simulink model "long"  (R2020a)
settings: Solver=VariableStepAuto  StartTime=0.0  StopTime=t_sim  MaxStep=0.01  RelTol=1e-3
values from neighbouring files (symbols this model uses):
  Cd0 = p_Cd(1)    [main.m]
  Cl0 = p_Cl(2)    [main.m]
  Cla = p_Cl(1)    [main.m]
  Cladot = pi + 2*pi*Gk/k    [main.m]
  Clde = Clde(1)    [main.m]
  Clq = -2*Cla*(h-3/4)    [main.m]
  Cm0 = p_Cm(2)    [main.m]
  Cma = p_Cm(1)    [main.m]
  Cmadot = pi*(h-1/2) + 2*pi*Gk/k*(h-1/4)    [main.m]
  Cmde = Clde(1)    [main.m]
  Cmq = -2*Cla*(h-1/2)^2    [main.m]
  delta_e = interp1(trim_polar(:,1),trim_polar(:,2),alpha)    [main.m]
  k = secante(func,0,1,1e-6,100)    [main.m]
  theta0 = 0    [main.m]
  u0 = tailsit.general.speed    [main.m]
  w0 = 0    [main.m]
undefined symbols (not defined in the file or in its folder): tailsit
libraries: simulink_extras x2
settings Model: Creator=willi  LastModifiedBy=willi
settings DataIOCC: ReturnWorkspaceOutputs=off
settings DebuggingCC: ArithmeticOperatorsInVariantConditions=warning
settings SFSimCC: SimUseLocalCustomCode=off  CustomCodeUndefinedFunction=UseInterfaceOnly
settings RTWCC: RTWUseLocalCustomCode=off

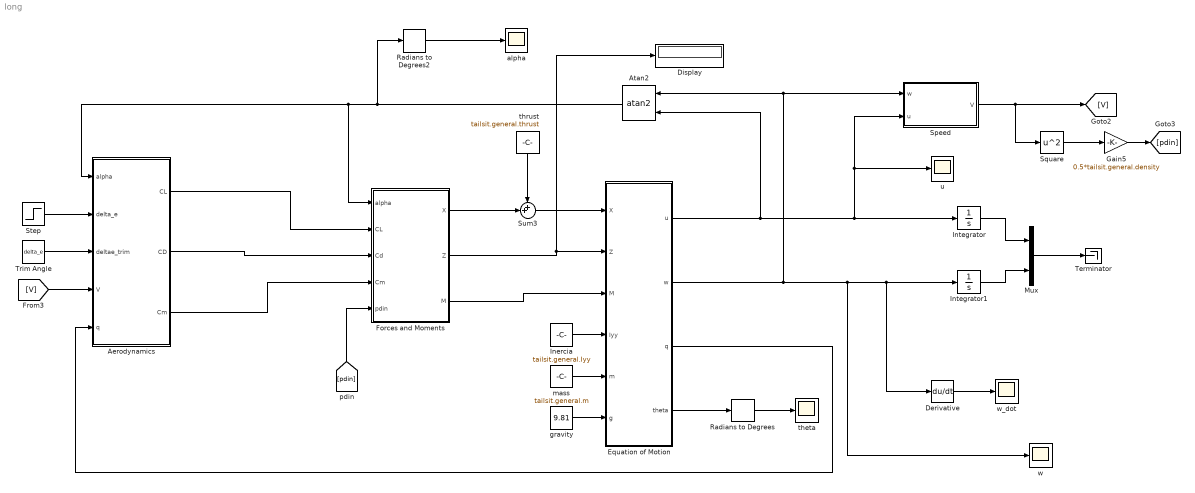
== system long ==
  Aerodynamics : Subsystem
  Atan2 : Trigonometry  Operator=atan2
  Derivative : Derivative
  Display : Display
  Equation of Motion : Subsystem  mask{initial_u=u0, initial_w=w0, initial_q=0.0, initial_theta=theta0}
      mask prompts: initial_u "Initial Speed (u, m/s)"; initial_w "Initial Speed (w, m/s)"; initial_q "Initial Angular Speed (q, rad/s)"; initial_theta "Euler Angle (theta, rad/s)"
  Forces and Moments : Subsystem  mask{area=tailsit.general.Sref, cref=tailsit.general.cbar}
      mask prompts: cref "Chord"
  Gain5 : Gain  Gain=0.5*tailsit.general.density
  Inercia : Constant  Value=tailsit.general.Iyy
  Integrator : Integrator
  Integrator1 : Integrator
  Mux : Mux  Inputs=2
  Radians to Degrees : simulink_extras/Transformations/Radians to Degrees
  Radians to Degrees2 : simulink_extras/Transformations/Radians to Degrees
  Speed : Subsystem
  Square : Math  Operator=square  SignedPower=on  SaturateOnIntegerOverflow=on
  Step : Step  Time=10  SampleTime=0
  Sum3 : Sum  Inputs=++|
  Terminator : Terminator
  Trim Angle : Constant  Value=delta_e
  alpha : Scope
  gravity : Constant  Value=9.81
  mass : Constant  Value=tailsit.general.m
  theta : Scope
  thrust : Constant  Value=tailsit.general.thrust
  u : Scope
  w : Scope
  w_dot : Scope
  wires:
  Forces and Moments/3(M) -> Equation of Motion/3(M)
  Forces and Moments/2(Z) -> Display/1, Equation of Motion/2(Z)
  Aerodynamics/1(CL) -> Forces and Moments/2(CL)
  thrust/1 -> Sum3/1
  Sum3/1 -> Equation of Motion/1(X)
  Forces and Moments/1(X) -> Sum3/2
  Equation of Motion/1(u) -> Integrator/1, Speed/2(u), u/1, Atan2/2
  Equation of Motion/2(w) -> Derivative/1, Integrator1/1, w/1, Speed/1("w "), Atan2/1
  Gain5/1 -> [pdin]
  [pdin] -> Forces and Moments/5(pdin)
  mass/1 -> Equation of Motion/5(m)
  gravity/1 -> Equation of Motion/6(g)
  Inercia/1 -> Equation of Motion/4(Iyy)
  Atan2/1 -> Radians to Degrees2/1, Aerodynamics/1(alpha), Forces and Moments/1(alpha)
  Radians to Degrees2/1 -> alpha/1
  Speed/1(V) -> [V], Square/1
  Square/1 -> Gain5/1
  Aerodynamics/2(CD) -> Forces and Moments/3(Cd)
  Aerodynamics/3(Cm) -> Forces and Moments/4(Cm)
  Trim Angle/1 -> Aerodynamics/3(deltae_trim)
  Equation of Motion/3(q) -> Aerodynamics/5(q)
  [V] -> Aerodynamics/4(V)
  Step/1 -> Aerodynamics/2(delta_e)
  Integrator/1 -> Mux/1
  Integrator1/1 -> Mux/2
  Mux/1 -> Terminator/1
  Derivative/1 -> w_dot/1
  Radians to Degrees/1 -> theta/1
  Equation of Motion/4(theta) -> Radians to Degrees/1

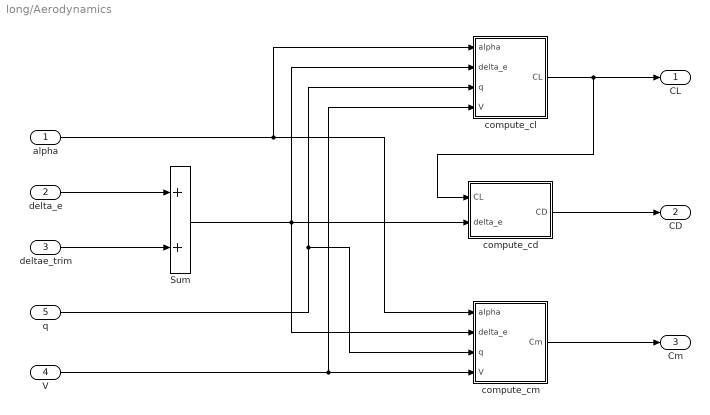
== system long/Aerodynamics ==
  alpha : Inport
  delta_e : Inport  Port=2
  deltae_trim : Inport  Port=3
  V : Inport  Port=4
  q : Inport  Port=5
  Sum : Sum
  compute_cd : Subsystem
  compute_cl : Subsystem
  compute_cm : Subsystem
  CL : Outport  VectorParamsAs1DForOutWhenUnconnected=off
  CD : Outport  Port=2  VectorParamsAs1DForOutWhenUnconnected=off
  Cm : Outport  Port=3  VectorParamsAs1DForOutWhenUnconnected=off
  wires:
  compute_cl/1(CL) -> compute_cd/1(CL), CL/1
  alpha/1 -> compute_cl/1(alpha), compute_cm/1(alpha)
  delta_e/1 -> Sum/1
  q/1 -> compute_cm/3(q), compute_cl/3(q)
  V/1 -> compute_cl/4(V), compute_cm/4(V)
  compute_cm/1(Cm) -> Cm/1
  compute_cd/1(CD) -> CD/1
  deltae_trim/1 -> Sum/2
  Sum/1 -> compute_cm/2(delta_e), compute_cl/2(delta_e), compute_cd/2(delta_e)

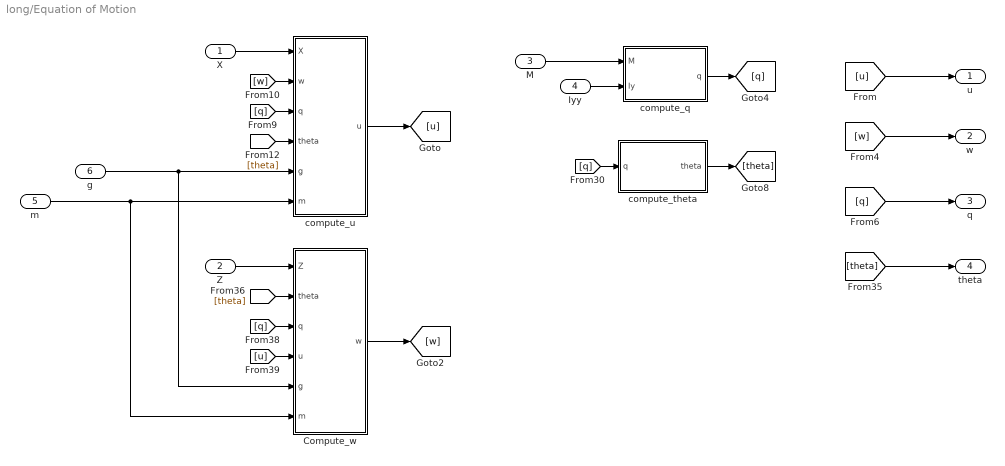
== system long/Equation of Motion ==
  X : Inport
  Z : Inport  Port=2
  M : Inport  Port=3
  Iyy : Inport  Port=4
  m : Inport  Port=5
  g : Inport  Port=6
  Compute_w : Subsystem
  compute_q : Subsystem
  compute_theta : Subsystem
  compute_u : Subsystem
  u : Outport  VectorParamsAs1DForOutWhenUnconnected=off
  w : Outport  Port=2  VectorParamsAs1DForOutWhenUnconnected=off
  q : Outport  Port=3  VectorParamsAs1DForOutWhenUnconnected=off
  theta : Outport  Port=4  VectorParamsAs1DForOutWhenUnconnected=off
  wires:
  X/1 -> compute_u/1(X)
  compute_u/1(u) -> [u]
  [u] -> u/1
  [w] -> w/1
  Z/1 -> Compute_w/1(Z)
  Compute_w/1(w) -> [w]
  M/1 -> compute_q/1(M)
  [q] -> q/1
  compute_q/1(q) -> [q]
  [w] -> compute_u/2(w)
  [q] -> compute_u/3(q)
  [theta] -> compute_u/4(theta)
  compute_theta/1("theta ") -> [theta]
  [q] -> compute_theta/1(q)
  [theta] -> theta/1
  [theta] -> Compute_w/2(theta)
  [q] -> Compute_w/3(q)
  [u] -> Compute_w/4(u)
  Iyy/1 -> compute_q/2(Iy)
  m/1 -> Compute_w/6(m), compute_u/6(m)
  g/1 -> Compute_w/5(g), compute_u/5(g)

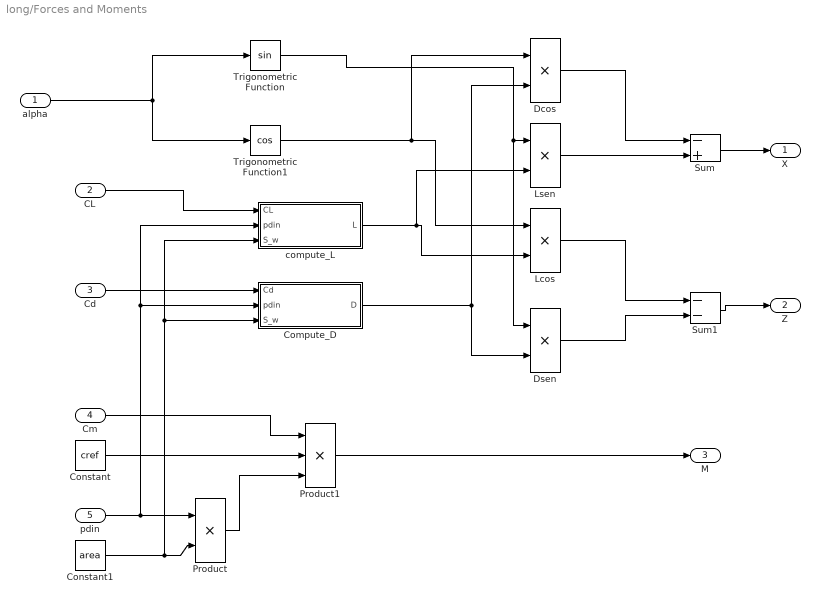
== system long/Forces and Moments ==
  alpha : Inport
  CL : Inport  Port=2
  Cd : Inport  Port=3
  Cm : Inport  Port=4
  pdin : Inport  Port=5
  Compute_D : Subsystem
  Constant : Constant  Value=cref
  Constant1 : Constant  Value=area
  Dcos : Product
  Dsen : Product
  Lcos : Product
  Lsen : Product
  Product : Product
  Product1 : Product  Inputs=3
  Sum : Sum  Inputs=-+
  Sum1 : Sum  Inputs=--
  Trigonometric Function : Trigonometry
  Trigonometric Function1 : Trigonometry  Operator=cos
  compute_L : Subsystem
  X : Outport  VectorParamsAs1DForOutWhenUnconnected=off
  Z : Outport  Port=2  VectorParamsAs1DForOutWhenUnconnected=off
  M : Outport  Port=3  VectorParamsAs1DForOutWhenUnconnected=off
  wires:
  Constant1/1 -> Compute_D/3(S_w), compute_L/3(S_w), Product/2
  Cm/1 -> Product1/1
  Constant/1 -> Product1/2
  Product/1 -> Product1/3
  Product1/1 -> M/1
  CL/1 -> compute_L/1(CL)
  Cd/1 -> Compute_D/1(Cd)
  pdin/1 -> Compute_D/2(pdin), compute_L/2(pdin), Product/1
  alpha/1 -> Trigonometric Function/1, Trigonometric Function1/1
  Sum/1 -> X/1
  Trigonometric Function1/1 -> Lcos/1, Dcos/1
  Compute_D/1(D) -> Dsen/2, Dcos/2
  compute_L/1(L) -> Lcos/2, Lsen/2
  Trigonometric Function/1 -> Dsen/1, Lsen/1
  Dcos/1 -> Sum/1
  Lsen/1 -> Sum/2
  Lcos/1 -> Sum1/1
  Dsen/1 -> Sum1/2
  Sum1/1 -> Z/1

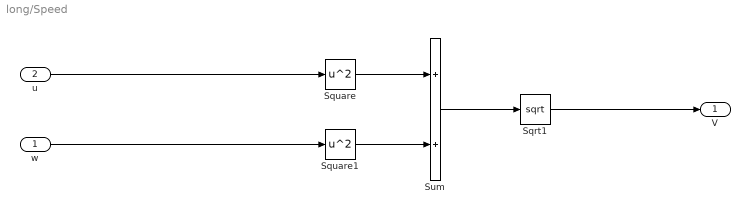
== system long/Speed ==
  "w " : Inport
  u : Inport  Port=2
  Sqrt1 : Sqrt  SaturateOnIntegerOverflow=on
  Square : Math  Operator=square  SignedPower=on  SaturateOnIntegerOverflow=on
  Square1 : Math  Operator=square  SignedPower=on  SaturateOnIntegerOverflow=on
  Sum : Sum
  V : Outport  VectorParamsAs1DForOutWhenUnconnected=off
  wires:
  Sum/1 -> Sqrt1/1
  Square1/1 -> Sum/2
  "w "/1 -> Square1/1
  Square/1 -> Sum/1
  u/1 -> Square/1
  Sqrt1/1 -> V/1

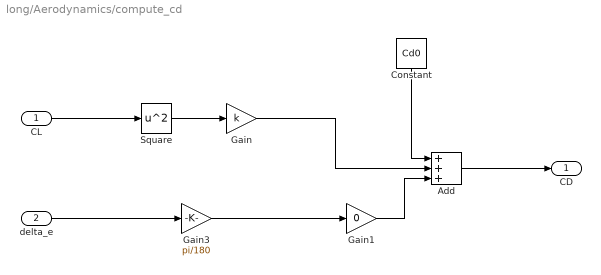
== system long/Aerodynamics/compute_cd ==
  CL : Inport
  delta_e : Inport  Port=2
  Add : Sum  Inputs=+++
  Constant : Constant  Value=Cd0
  Gain : Gain  Gain=k
  Gain1 : Gain  Gain=0
  Gain3 : Gain  Gain=pi/180
  Square : Math  Operator=square  SignedPower=on  SaturateOnIntegerOverflow=on
  CD : Outport  VectorParamsAs1DForOutWhenUnconnected=off
  wires:
  Add/1 -> CD/1
  Gain1/1 -> Add/3
  Constant/1 -> Add/1
  CL/1 -> Square/1
  delta_e/1 -> Gain3/1
  Gain3/1 -> Gain1/1
  Square/1 -> Gain/1
  Gain/1 -> Add/2

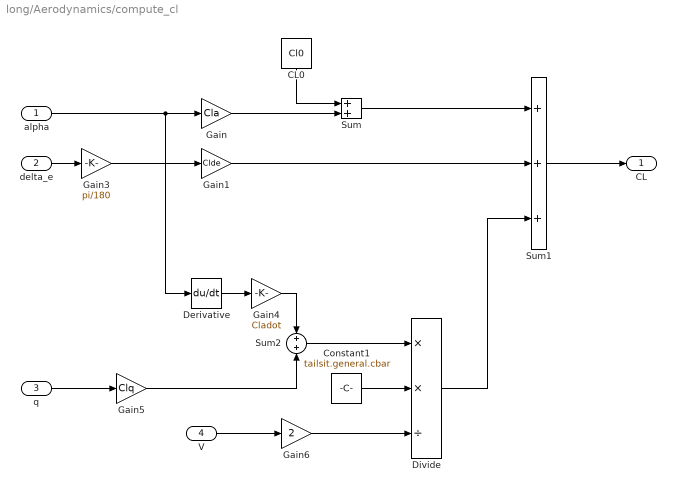
== system long/Aerodynamics/compute_cl ==
  alpha : Inport
  delta_e : Inport  Port=2
  q : Inport  Port=3
  V : Inport  Port=4
  CL0 : Constant  Value=Cl0
  Constant1 : Constant  Value=tailsit.general.cbar
  Derivative : Derivative
  Divide : Product  Inputs=**/
  Gain : Gain  Gain=Cla
  Gain1 : Gain  Gain=Clde
  Gain3 : Gain  Gain=pi/180
  Gain4 : Gain  Gain=Cladot
  Gain5 : Gain  Gain=Clq
  Gain6 : Gain  Gain=2
  Sum : Sum
  Sum1 : Sum  Inputs=+++
  Sum2 : Sum
  CL : Outport  VectorParamsAs1DForOutWhenUnconnected=off
  wires:
  CL0/1 -> Sum/1
  Gain/1 -> Sum/2
  Sum/1 -> Sum1/1
  Gain1/1 -> Sum1/2
  alpha/1 -> Derivative/1, Gain/1
  delta_e/1 -> Gain3/1
  Gain3/1 -> Gain1/1
  Derivative/1 -> Gain4/1
  Gain4/1 -> Sum2/1
  q/1 -> Gain5/1
  Gain5/1 -> Sum2/2
  Sum1/1 -> CL/1
  V/1 -> Gain6/1
  Sum2/1 -> Divide/1
  Constant1/1 -> Divide/2
  Gain6/1 -> Divide/3
  Divide/1 -> Sum1/3

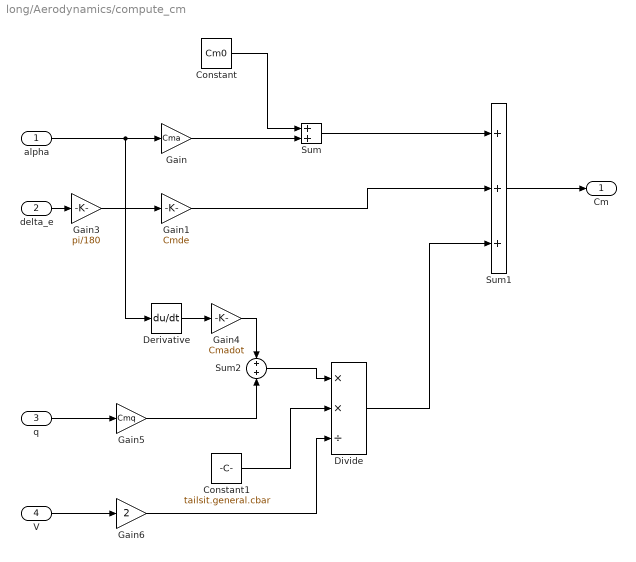
== system long/Aerodynamics/compute_cm ==
  alpha : Inport
  delta_e : Inport  Port=2
  q : Inport  Port=3
  V : Inport  Port=4
  Constant : Constant  Value=Cm0
  Constant1 : Constant  Value=tailsit.general.cbar
  Derivative : Derivative
  Divide : Product  Inputs=**/
  Gain : Gain  Gain=Cma
  Gain1 : Gain  Gain=Cmde
  Gain3 : Gain  Gain=pi/180
  Gain4 : Gain  Gain=Cmadot
  Gain5 : Gain  Gain=Cmq
  Gain6 : Gain  Gain=2
  Sum : Sum
  Sum1 : Sum  Inputs=+++
  Sum2 : Sum
  Cm : Outport  VectorParamsAs1DForOutWhenUnconnected=off
  wires:
  Constant/1 -> Sum/1
  Gain/1 -> Sum/2
  Sum/1 -> Sum1/1
  Gain1/1 -> Sum1/2
  alpha/1 -> Derivative/1, Gain/1
  delta_e/1 -> Gain3/1
  Gain3/1 -> Gain1/1
  Derivative/1 -> Gain4/1
  Gain4/1 -> Sum2/1
  q/1 -> Gain5/1
  Gain5/1 -> Sum2/2
  Divide/1 -> Sum1/3
  Sum1/1 -> Cm/1
  Sum2/1 -> Divide/1
  V/1 -> Gain6/1
  Gain6/1 -> Divide/3
  Constant1/1 -> Divide/2

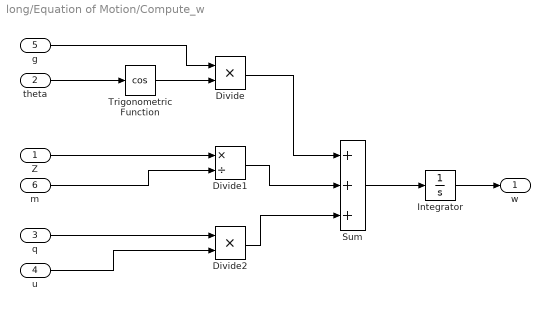
== system long/Equation of Motion/Compute_w ==
  Z : Inport
  theta : Inport  Port=2
  q : Inport  Port=3
  u : Inport  Port=4
  g : Inport  Port=5
  m : Inport  Port=6
  Divide : Product  Inputs=**
  Divide1 : Product  Inputs=*/
  Divide2 : Product  Inputs=**
  Integrator : Integrator
  Sum : Sum  Inputs=+++
  Trigonometric Function : Trigonometry  Operator=cos
  w : Outport  VectorParamsAs1DForOutWhenUnconnected=off
  wires:
  Integrator/1 -> w/1
  u/1 -> Divide2/2
  Sum/1 -> Integrator/1
  m/1 -> Divide1/2
  Trigonometric Function/1 -> Divide/2
  Divide2/1 -> Sum/3
  Z/1 -> Divide1/1
  Divide1/1 -> Sum/2
  theta/1 -> Trigonometric Function/1
  Divide/1 -> Sum/1
  q/1 -> Divide2/1
  g/1 -> Divide/1

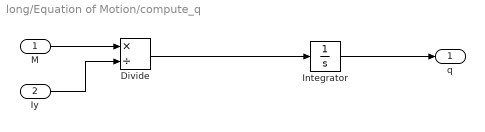
== system long/Equation of Motion/compute_q ==
  M : Inport
  Iy : Inport  Port=2
  Divide : Product  Inputs=*/
  Integrator : Integrator  InitialCondition=initial_q
  q : Outport  VectorParamsAs1DForOutWhenUnconnected=off
  wires:
  M/1 -> Divide/1
  Iy/1 -> Divide/2
  Divide/1 -> Integrator/1
  Integrator/1 -> q/1

== system long/Equation of Motion/compute_theta ==
  q : Inport
  Integrator : Integrator  InitialCondition=initial_theta
  "theta " : Outport  VectorParamsAs1DForOutWhenUnconnected=off
  wires:
  q/1 -> Integrator/1
  Integrator/1 -> "theta "/1

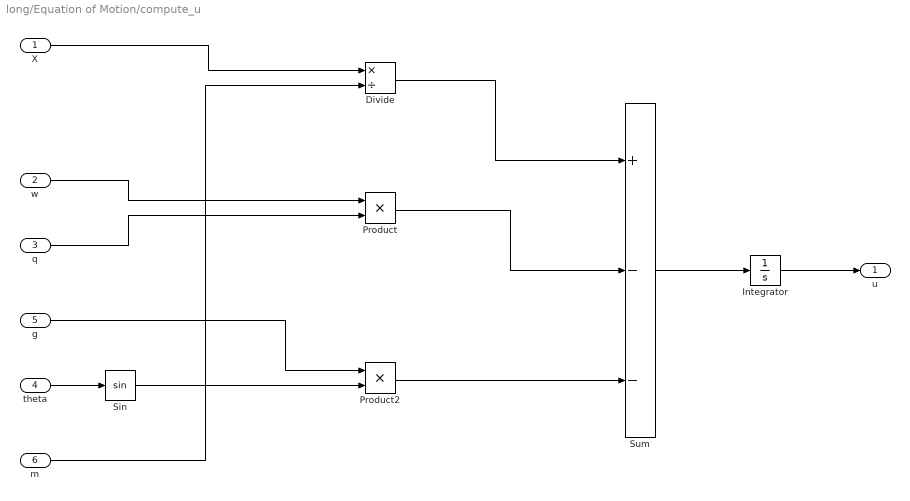
== system long/Equation of Motion/compute_u ==
  X : Inport
  w : Inport  Port=2
  q : Inport  Port=3
  theta : Inport  Port=4
  g : Inport  Port=5
  m : Inport  Port=6
  Divide : Product  Inputs=*/
  Integrator : Integrator  InitialCondition=initial_u
  Product : Product
  Product2 : Product
  Sin : Trigonometry
  Sum : Sum  Inputs=+--
  u : Outport  VectorParamsAs1DForOutWhenUnconnected=off
  wires:
  X/1 -> Divide/1
  m/1 -> Divide/2
  q/1 -> Product/2
  w/1 -> Product/1
  theta/1 -> Sin/1
  Sin/1 -> Product2/2
  g/1 -> Product2/1
  Divide/1 -> Sum/1
  Product2/1 -> Sum/3
  Product/1 -> Sum/2
  Sum/1 -> Integrator/1
  Integrator/1 -> u/1

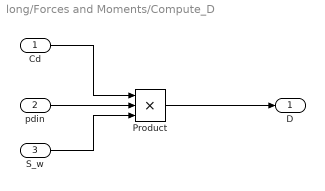
== system long/Forces and Moments/Compute_D ==
  Cd : Inport
  pdin : Inport  Port=2
  S_w : Inport  Port=3
  Product : Product  Inputs=3
  D : Outport  VectorParamsAs1DForOutWhenUnconnected=off
  wires:
  Cd/1 -> Product/1
  pdin/1 -> Product/2
  S_w/1 -> Product/3
  Product/1 -> D/1

== system long/Forces and Moments/compute_L ==
  CL : Inport
  pdin : Inport  Port=2
  S_w : Inport  Port=3
  Product : Product  Inputs=3
  L : Outport  VectorParamsAs1DForOutWhenUnconnected=off
  wires:
  CL/1 -> Product/1
  pdin/1 -> Product/2
  S_w/1 -> Product/3
  Product/1 -> L/1
